simulink model "lab64"  (R2023b)
settings: Solver=VariableStepAuto  StartTime=0.0  StopTime=20  RelTol=1e-3
undefined symbols (not defined in the file or in its folder): kp_PWM2
settings Model: Creator=Настя  LastModifiedBy=killer
settings SolverCC: AlgebraicLoopSolver=TrustRegion
settings DebuggingCC: UnconnectedInputMsg=warning  UnconnectedOutputMsg=warning  UnconnectedLineMsg=warning
settings ModelReferenceCC: EnableRefExpFcnMdlSchedulingChecks=on
settings RTWCC: DLArmComputeVersion=19.05

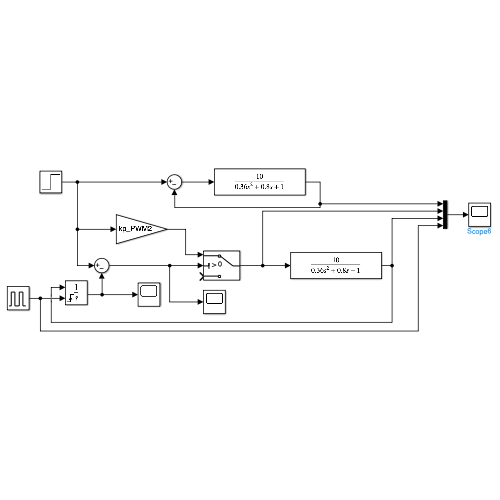
[thumbnail: Simulink's stored preview of the top-level diagram]
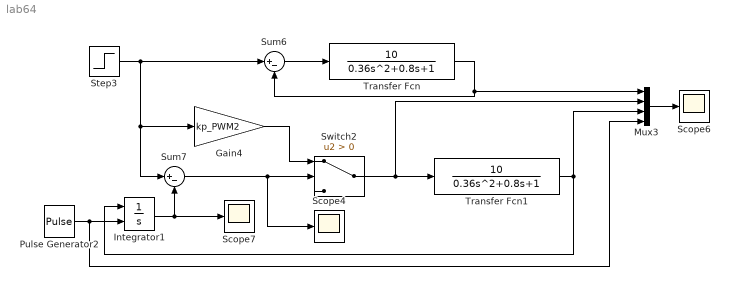
== system lab64 ==
  Gain4 : Gain  Gain=kp_PWM2
  Integrator1 : Integrator  ExternalReset=rising
  Mux3 : Mux
  Pulse Generator2 : DiscretePulseGenerator  PulseType=Time based  Amplitude=0.1  Period=0.5  PulseWidth=0.02
  Scope4 : Scope
  Scope6 : Scope
  Scope7 : Scope
  Step3 : Step  Time=0  SampleTime=0
  Sum6 : Sum  Inputs=|+-
  Sum7 : Sum  Inputs=|+-
  Switch2 : Switch  Criteria=u2 > Threshold  SaturateOnIntegerOverflow=off  InputSameDT=off
  Transfer Fcn : TransferFcn  Numerator=[10]  Denominator=[0.36 0.8 1]
  Transfer Fcn1 : TransferFcn  Numerator=[10]  Denominator=[0.36 0.8 1]
  wires:
  Switch2/1 -> Transfer Fcn1/1, Mux3/2
  Sum6/1 -> Transfer Fcn/1
  Sum7/1 -> Scope4/1, Switch2/2
  Integrator1/1 -> Sum7/2, Scope7/1
  Pulse Generator2/1 -> Mux3/4, Integrator1/2
  Mux3/1 -> Scope6/1
  Gain4/1 -> Switch2/1
  Transfer Fcn/1 -> Sum6/2, Mux3/1
  Transfer Fcn1/1 -> Mux3/3, Integrator1/1
  Step3/1 -> Sum7/1, Gain4/1, Sum6/1
